simulink model "P1_Ex1"  (R2018a)
settings: Solver=FixedStepAuto  StartTime=0.0  StopTime=40  RelTol=1e-3  EnableMultiTasking=on
PreLoadFcn:
  | % Sampling times
  | Tg=0.005;
  | Ts=0.01;
  | % Motor limits
  | Vmax=5;
  | Vmin=-5;
  | % Proportional controller's gain
  | Kp=1;
libraries: arduinolib x4
settings Model: SimulationMode=external  ExtModeTrigDuration=2  Creator=Eneko Lerma  LastModifiedBy=Eneko Lerma
settings SolverCC: AutoInsertRateTranBlk=on
settings OptimizationCC: EnhancedBackFolding=on  PassReuseOutputArgsAs=Individual arguments  MaxStackSize=64  OptimizeBlockOrder=speed  DifferentSizesBufferReuse=on  OptimizationCustomize=off
settings DebuggingCC: ParameterPrecisionLossMsg=none  ParameterTunabilityLossMsg=error
settings HardwareCC: ProdBitPerPointer=32  ProdBitPerSizeT=32  ProdBitPerPtrDiffT=32  ProdLargestAtomicInteger=Long  ProdLargestAtomicFloat=Double  ProdWordSize=32  ProdHWDeviceType=ARM Compatible->ARM Cortex
settings SFSimCC: MATLABDynamicMemAlloc=off
settings RTWCC: SystemTargetFile=ert.tlc  HardwareBoard=Arduino Due  TLCOptions=-aInlineSetEventsForThisBaseRateFcn=TLC_FALSE -aSuppressMultiTaskScheduler=TLC_FALSE -aRateBasedStepFcn=1  TemplateMakefile=ert_default_tmf  GenerateReport=on  Toolchain=Arduino ARM  BuildConfiguration=Faster Runs  IncludeHyperlinkInReport=on  LaunchReport=on  GenerateTraceInfo=on  GenerateTraceReport=on  GenerateTraceReportSl=on  GenerateTraceReportSf=on  GenerateTraceReportEml=on
settings RTWCC: CustomTerminator=|
  | writeDigitalPin((uint8_T)3, 0);
  | writeDigitalPin((uint8_T)5, 0);
settings CodeAppCC: ForceParamTrailComments=on  IgnoreCustomStorageClasses=off  OperatorAnnotations=on  SimulinkDataObjDesc=on  SFDataObjDesc=on  InsertBlockDesc=on
settings ERTTargetCC: SupportContinuousTime=on  SupportVariableSizeSignals=on

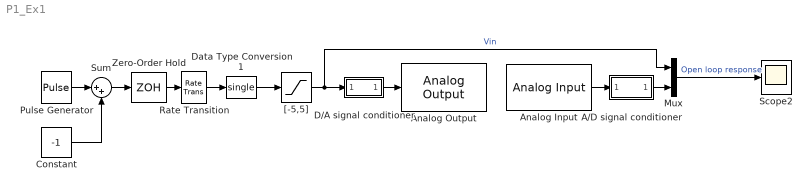
== system P1_Ex1 ==
  A/D signal conditioner : Subsystem
  Analog Input : arduinolib/Analog Input  pinNumber=0  ReadResultsOnly=off  ConversionTriggerSource=Software  ExternalTriggerType=uint32(0)  OutputDataType=uint16  EnableConversionCompleteNotify=off  EnableOuputStatus=off  SampleTime=Tg  blockPlatform=arduino
  Analog Output : arduinolib/Analog Output  DACpin=DAC1  blockPlatform=arduino
      settings: SourceProductName=Simulink Support Package for Arduino Hardware  SourceProductBaseCode=ARDUINO
  Constant : Constant  Value=-1
  D/A signal conditioner : Subsystem
  Data Type Conversion1 : DataTypeConversion  OutDataTypeStr=single
  Mux : Mux  Inputs=2
  Pulse Generator : DiscretePulseGenerator  PulseType=Time based  Amplitude=2  Period=10  PulseWidth=50  SampleTime=0.005
  Rate Transition : RateTransition
  Scope2 : Scope
  Sum : Sum  Inputs=|++
  Zero-Order Hold : ZeroOrderHold  SampleTime=Ts
  "[-5,5]" : Saturate  UpperLimit=Vmax  LowerLimit=Vmin  OutDataTypeStr=single
  wires:
  Mux/1 -> Scope2/1  "Open loop response"
  "[-5,5]"/1 -> Mux/1, D/A signal conditioner/1("  ")  "Vin"
  D/A signal conditioner/1(" ") -> Analog Output/1
  Analog Input/1 -> A/D signal conditioner/1(" ")
  A/D signal conditioner/1(" ") -> Mux/2
  Data Type Conversion1/1 -> "[-5,5]"/1
  Zero-Order Hold/1 -> Rate Transition/1
  Pulse Generator/1 -> Sum/1
  Sum/1 -> Zero-Order Hold/1
  Constant/1 -> Sum/2
  Rate Transition/1 -> Data Type Conversion1/1

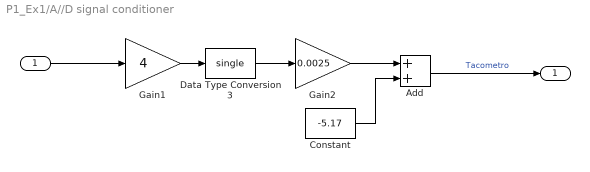
== system P1_Ex1/A//D signal conditioner ==
  " " : Inport
  Add : Sum  AccumDataTypeStr=single
  Constant : Constant  Value=-5.17  OutDataTypeStr=single
  Data Type Conversion3 : DataTypeConversion  OutDataTypeStr=single
  Gain1 : Gain  Gain=4  OutDataTypeStr=uint16
  Gain2 : Gain  Gain=0.0025  OutDataTypeStr=single
  " " : Outport
  wires:
  Gain1/1 -> Data Type Conversion3/1
  " "/1 -> Gain1/1
  Add/1 -> " "/1  "Tacometro"
  Gain2/1 -> Add/1
  Constant/1 -> Add/2
  Data Type Conversion3/1 -> Gain2/1

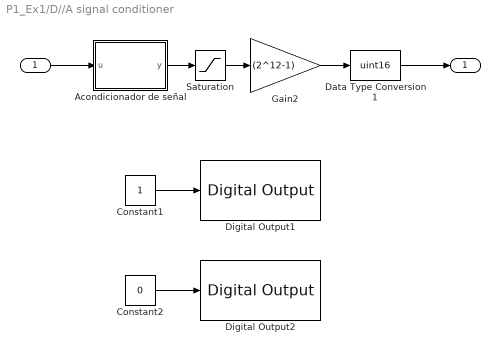
== system P1_Ex1/D//A signal conditioner ==
  "  " : Inport  OutDataTypeStr=single
  Acondicionador de señal : MATLAB Function  TreatAsAtomicUnit=on
  Constant1 : Constant
  Constant2 : Constant  Value=0
  Data Type Conversion1 : DataTypeConversion  OutDataTypeStr=uint16
  Digital Output1 : arduinolib/Digital Output  pinNumber=5  blockPlatform=arduino
  Digital Output2 : arduinolib/Digital Output  pinNumber=3  blockPlatform=arduino
  Gain2 : Gain  Gain=(2^12-1)  OutDataTypeStr=single
  Saturation : Saturate  UpperLimit=1  LowerLimit=0  OutDataTypeStr=single
  " " : Outport  OutDataTypeStr=uint16
  wires:
  Saturation/1 -> Gain2/1
  Data Type Conversion1/1 -> " "/1
  Acondicionador de señal/1(y) -> Saturation/1
  "  "/1 -> Acondicionador de señal/1(u)
  Gain2/1 -> Data Type Conversion1/1
  Constant2/1 -> Digital Output2/1
  Constant1/1 -> Digital Output1/1

== matlab function P1_Ex1/D//A signal conditioner/Acondicionador de señal ==
  data: u input; y output
function y = fcn(u)
y =0.0968*u+0.5085;
